simulink model "lab3p2"  (R2019a)
settings: Solver=VariableStepAuto  StartTime=0.0  StopTime=10  RelTol=1e-3
settings Model: Creator=sk  LastModifiedBy=sk

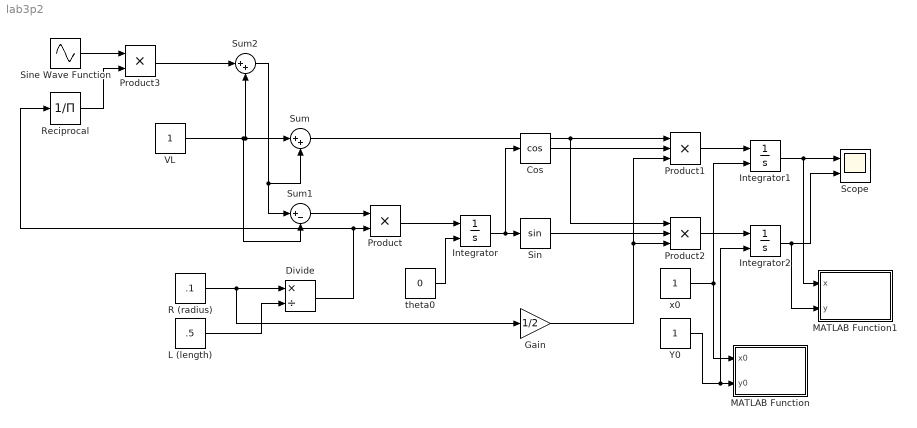
== system lab3p2 ==
  Cos : Trigonometry  Operator=cos
  Divide : Product  Inputs=*/
  Gain : Gain  Gain=1/2
  Integrator : Integrator  InitialConditionSource=external
  Integrator1 : Integrator  InitialConditionSource=external
  Integrator2 : Integrator  InitialConditionSource=external
  L (length) : Constant  Value=.5
  MATLAB Function : MATLAB Function  TreatAsAtomicUnit=on
  MATLAB Function1 : MATLAB Function  TreatAsAtomicUnit=on
  Product : Product
  Product1 : Product  Inputs=3
  Product2 : Product  Inputs=3
  Product3 : Product
  R (radius) : Constant  Value=.1
  Reciprocal : Product  Inputs=/
  Scope : Scope  NumInputPorts=2
  Sin : Trigonometry
  Sine Wave Function : Sin  Frequency=100  SampleTime=0
  Sum : Sum  Inputs=|++
  Sum1 : Sum  Inputs=|+-
  Sum2 : Sum  Inputs=|++
  VL : Constant
  "Y0 " : Constant
  "theta0 " : Constant  Value=0
  "x0 " : Constant
  wires:
  VL/1 -> Sum2/2, Sum/1, Sum1/2
  Sum2/1 -> Sum1/1, Sum/2
  R (radius)/1 -> Gain/1, Divide/1
  L (length)/1 -> Divide/2
  Sum1/1 -> Product/1
  Divide/1 -> Reciprocal/1, Product/2
  Product/1 -> Integrator/1
  "theta0 "/1 -> Integrator/2
  Integrator/1 -> Cos/1, Sin/1
  Cos/1 -> Product1/2
  Gain/1 -> Product2/3, Product1/3
  Sin/1 -> Product2/2
  Sum/1 -> Product2/1, Product1/1
  Product1/1 -> Integrator1/1
  Product2/1 -> Integrator2/1
  "x0 "/1 -> MATLAB Function/1(x0), Integrator1/2
  "Y0 "/1 -> Integrator2/2, MATLAB Function/2(y0)
  Integrator2/1 -> MATLAB Function1/2(y), Scope/2
  Integrator1/1 -> MATLAB Function1/1(x), Scope/1
  Sine Wave Function/1 -> Product3/1
  Reciprocal/1 -> Product3/2
  Product3/1 -> Sum2/1

== matlab function lab3p2/MATLAB Function1 ==
  data: x input; y input
function fcn(x,y)
plot(x,y,'*b')
end

== matlab function lab3p2/MATLAB Function ==
  data: x0 input; y0 input
function fcn(x0,y0)
plot(x0,y0,'*r')
hold on
end
